simulink model "sis_pendolo_ctrl_oss"  (Simulink 7.6)
settings: Solver=ode45  StartTime=0.0  StopTime=10.0  RelTol=1e-3
values from neighbouring files (symbols this model uses):
  F1 = 1    [pendolo_own.m]
  F2 = 0    [pendolo_own.m]
  h = 0.2    [pendolo_own.m]
  J = m*L^2    (= 1)    [pendolo_own.m]
  L = 1    [pendolo_own.m]
  x0 = [.1 0]'    [pendolo_own.m]
libraries: simulink x1
settings Model: Creator=professore  LastModifiedBy=patrizio

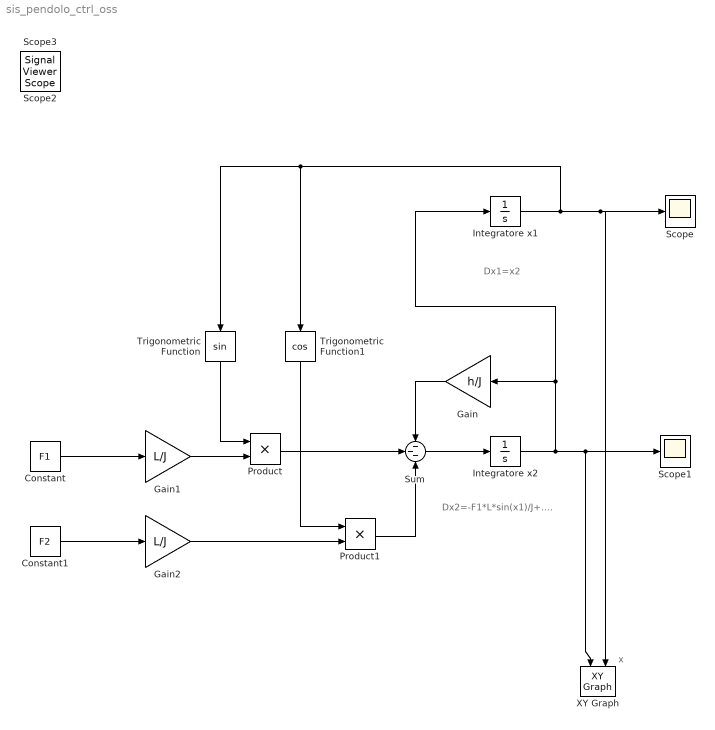
== system sis_pendolo_ctrl_oss ==
  note: x
  note: Dx1=x2
  note: Dx2=-F1*L*sin(x1)/J+....
  Constant : Constant  Value=F1
  Constant1 : Constant  Value=F2
  Gain : Gain  Gain=h/J
  Gain1 : Gain  Gain=L/J
  Gain2 : Gain  Gain=L/J
  Integratore x1 : Integrator  InitialCondition=x0(1)
  Integratore x2 : Integrator  InitialCondition=x0(2)
  Product : Product  RndMeth=Zero
  Product1 : Product  RndMeth=Zero
  Scope : Scope
  Scope1 : Scope
  Sum : Sum  Inputs=---
  Trigonometric Function : Trigonometry
  Trigonometric Function1 : Trigonometry  Operator=cos
  XY Graph : simulink/Sinks/XY Graph  SystemSampleTime=-1  xmin=-1  xmax=1  ymin=-1  ymax=1  st=-1
  Scope2 : SignalViewerScope  IOType=viewer  RefreshTime=0.035000
  Scope3 : SignalViewerScope  IOType=viewer  RefreshTime=0.035000
  wires:
  Sum/1 -> Integratore x2/1
  Integratore x2/1 -> Integratore x1/1, Gain/1, Scope1/1, XY Graph/1
  Gain/1 -> Sum/1
  Gain1/1 -> Product/2
  Product/1 -> Sum/2
  Constant/1 -> Gain1/1
  Gain2/1 -> Product1/2
  Product1/1 -> Sum/3
  Trigonometric Function1/1 -> Product1/1
  Trigonometric Function/1 -> Product/1
  Constant1/1 -> Gain2/1
  Integratore x1/1 -> Trigonometric Function/1, Trigonometric Function1/1, Scope/1, XY Graph/2
